simulink model "modele"  (R2016a)
settings: Solver=VariableStepAuto  StartTime=0.0  StopTime=10.0  RelTol=1e-3
settings Model: Creator=nizar  LastModifiedBy=nizar

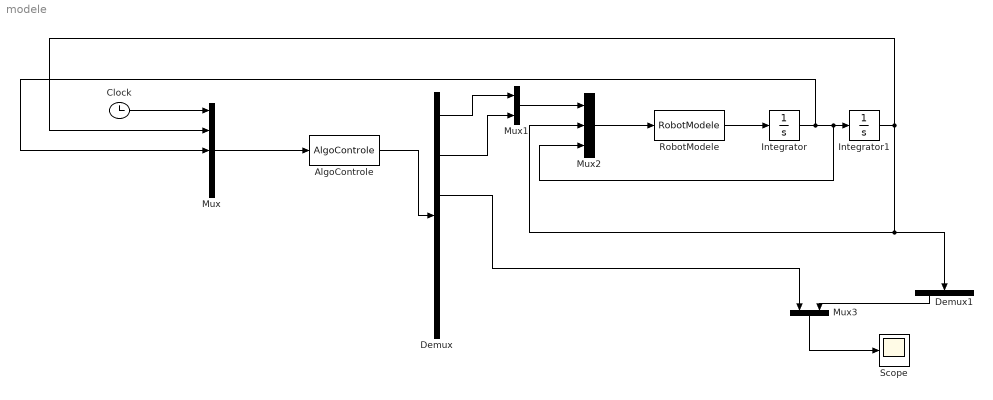
== system modele ==
  AlgoControle : MATLABFcn  MATLABFcn=AlgoControle  OutputDimensions=6
  Clock : Clock
  Demux : Demux  Outputs=6
  Demux1 : Demux  Outputs=2
  Integrator : Integrator
  Integrator1 : Integrator
  Mux : Mux  Inputs=5
  Mux1 : Mux  Inputs=2
  Mux2 : Mux  Inputs=3
  Mux3 : Mux  Inputs=2
  RobotModele : MATLABFcn  MATLABFcn=RobotModele  OutputDimensions=2
  Scope : Scope
  wires:
  Clock/1 -> Mux/1
  Mux/1 -> AlgoControle/1
  AlgoControle/1 -> Demux/1
  Demux/1 -> Mux1/1
  Demux/2 -> Mux1/2
  Mux1/1 -> Mux2/1
  Mux2/1 -> RobotModele/1
  RobotModele/1 -> Integrator/1
  Integrator/1 -> Mux/3, Mux2/3, Integrator1/1
  Integrator1/1 -> Mux2/2, Demux1/1, Mux/2
  Mux3/1 -> Scope/1
  Demux/3 -> Mux3/1
  Demux1/1 -> Mux3/2
